simulink model "filtering"  (R2024a)
settings: Solver=FixedStepAuto  StartTime=0.0  StopTime=inf  FixedStep=1e-3  RelTol=1e-3
values from neighbouring files (symbols this model uses):
  net = trainNetwork(XTrain, YTrain, layers, options)    [lstm_ex.m]    (also in optimization.m; simpleCanvas.m)
undefined symbols (not defined in the file or in its folder): CR, LF
libraries: dspstat3 x5, instrumentseriallib x2, dspfdesign x1, deeplib x1
settings Model: Creator=samet  LastModifiedBy=samet
settings OptimizationCC: BlockReduction=off  DefaultParameterBehavior=Inlined  BufferReuse=off

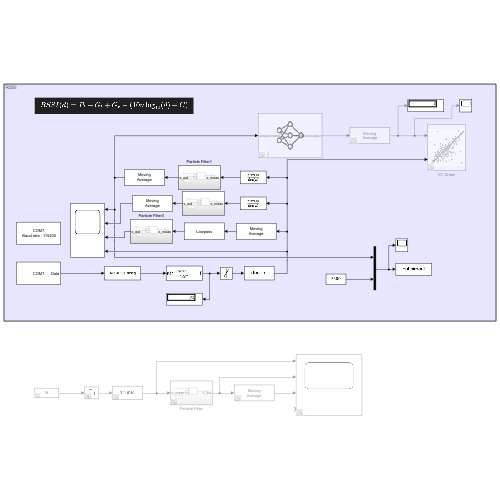
[thumbnail: Simulink's stored preview of the top-level diagram]
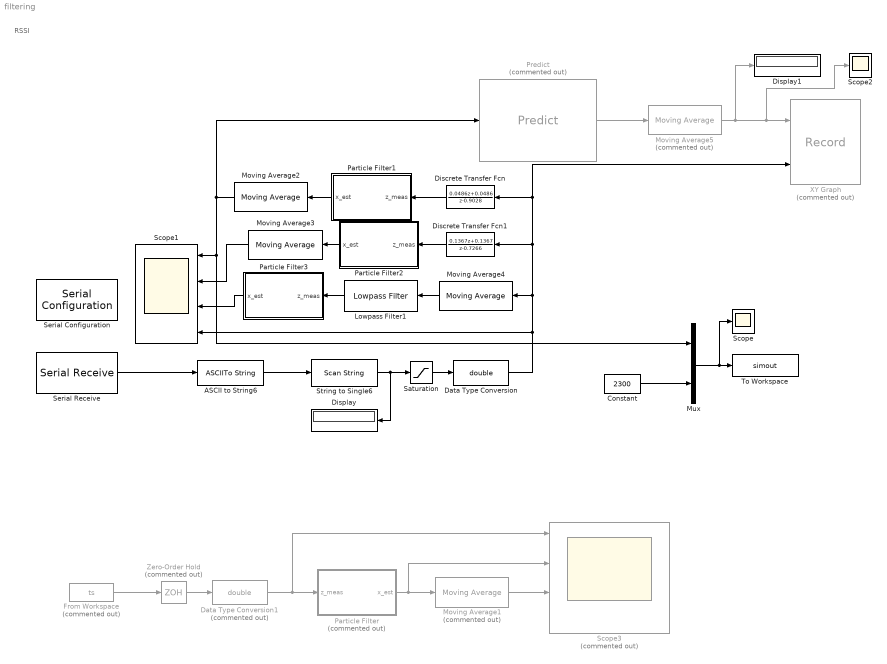
== system filtering ==
  note: RSSI
  ASCII to String6 : ASCIIToString
  Constant : Constant  Value=2300
  Data Type Conversion : DataTypeConversion  OutDataTypeStr=double  SaturateOnIntegerOverflow=off  RndMeth=Floor
  Data Type Conversion1 : DataTypeConversion  Commented=on  OutDataTypeStr=double  SaturateOnIntegerOverflow=off  RndMeth=Floor
  Discrete Transfer Fcn : DiscreteTransferFcn  Numerator=[0.0486 0.0486]  Denominator=[1 -0.9028]
  Discrete Transfer Fcn1 : DiscreteTransferFcn  Numerator=[0.1367 0.1367]  Denominator=[1 -0.7266]
  Display : Display
  Display1 : Display
  From Workspace : FromWorkspace  Commented=on  VariableName=ts
  Lowpass Filter1 : dspfdesign/Lowpass Filter  FilterType=FIR  DesignForMinimumOrder=on  FilterOrder=50  PassbandFrequency=8e3  StopbandFrequency=12e3  PassbandRipple=0.1  StopbandAttenuation=1  SampleRateMode=Specify on dialog  SampleRate=44100  SimulateUsing=Interpreted execution  roundingMode=Floor  coeffsDataTypeStr=fixdt(1,16)
  Moving Average1 : dspstat3/Moving Average  Commented=on  Method=Sliding window  ForgettingFactorPort=off  SpecifyWindowLength=on  WindowLength=4  OverlapLength=3  AllowArbitraryInputLength=off  ForgettingFactor=0.9  SimulateUsing=Interpreted execution
  Moving Average2 : dspstat3/Moving Average  Method=Sliding window  ForgettingFactorPort=off  SpecifyWindowLength=on  WindowLength=12  OverlapLength=11  AllowArbitraryInputLength=off  ForgettingFactor=0.9  SimulateUsing=Interpreted execution
  Moving Average3 : dspstat3/Moving Average  Method=Sliding window  ForgettingFactorPort=off  SpecifyWindowLength=on  WindowLength=12  OverlapLength=11  AllowArbitraryInputLength=off  ForgettingFactor=0.9  SimulateUsing=Interpreted execution
  Moving Average4 : dspstat3/Moving Average  Method=Sliding window  ForgettingFactorPort=off  SpecifyWindowLength=on  WindowLength=4  OverlapLength=3  AllowArbitraryInputLength=off  ForgettingFactor=0.9  SimulateUsing=Interpreted execution
  Moving Average5 : dspstat3/Moving Average  Commented=on  Method=Sliding window  ForgettingFactorPort=off  SpecifyWindowLength=on  WindowLength=12  OverlapLength=11  AllowArbitraryInputLength=off  ForgettingFactor=0.9  SimulateUsing=Interpreted execution
  Mux : Mux  Inputs=2
  Particle Filter : Subsystem  Commented=on
  Particle Filter1 : Subsystem
  Particle Filter2 : Subsystem
  Particle Filter3 : Subsystem
  Predict : deeplib/Predict  Commented=on  Network=Network from MAT-file  NetworkFunction=squeezenet  NetworkFilePath=C:\Users\samet\Desktop\net.mat  MiniBatchSize=128  InputDataFormats={'',''}  Predictions=on  Activations={}  ForceInterpretedSim=off  EnableDLNetwork=on  LastKnownNetworkFilePath=''  LastKnownNetworkTimeStamp=''
  Saturation : Saturate  UpperLimit=0  LowerLimit=-80
  Scope : Scope
  Scope1 : Scope  NumInputPorts=4
  Scope2 : Scope
  Scope3 : Scope  Commented=on  NumInputPorts=4
  Serial Configuration : instrumentseriallib/Serial Configuration  Priority=-200000  PortSel=COM7  Port=COM7  ComPort=COM7  BaudRate=115200  DataBits=8  Parity=none  StopBits=1  ByteOrder=little-endian  FlowControl=none  Timeout=10  SimulateUsing=Interpreted execution  BlockInModel=on  aMode=1
      settings: LibrarySourceBlock=embeddedtargetslib/Host Communication/Serial Configuration
  Serial Receive : instrumentseriallib/Serial Receive  Priority=1  PortSel=COM7  Port=COM7  ComPort=COM7  DataType=uint8  SaveDataType=uint8  ToggleHeader=off  Header=[]  ToggleDataSize=on  DataSize=[1 3]  ToggleTerminator=on  Terminator=CR/LF ('\r\n')  CustomTerminator='\n\r'  InputFormat=Row major  EnableBlockingMode=on  ActionDataUnavailable=Output last received value  ActionWhenDataUnavailable=Output last received value  CustomValue=0  SampleTime=0.01  SimulateUsing=Interpreted execution  BlockInModel=on  aMode=1
      settings: LibrarySourceBlock=embeddedtargetslib/Host Communication/Serial Receive
  String to Single6 : ScanString  Format="\"%f\""
  To Workspace : ToWorkspace  VariableName=simout  SampleTime=-1
      settings: Save2DSignal=2-D array (concatenate along first dimension)
  XY Graph : Record  Commented=on  FileSettingsInternal="{\"entries\":[{\"content\":{\"excelSettings\":{\"content\":{},\"type\":\"Streamout.ExcelSettings\"}},\"type\":\"Streamout.FileSettingStorage\",\"uuid\":\"\"}],\"packageUris\":[\"http:\\/\\/schema.mathworks.com\\/mf0\\/streamout_blocks\\/R2020a\"],\"version\":\"1.0\"}"  Layout=[1 1]  SignalsInternal="{\"entries\":[{\"content\":{\"signals\":[{\"content\":{\"blockPath\":[],\"dimensions\":[1,1],\"domain\":\"\",\"lineColor\":\"#22b573\",\"lineWidth\":2,\"port\":1,\"signalID\":1,\"signalName\":\"Moving\\nAverage5\"},\"type\":\"RecordBlkView.Signal\",\"uuid\":\"\"},{\"content\":{\"blockPath\":[],\"dimensions\":[1],\"domain\":\"\",\"lineColor\":\"#0072bd\",\"lineWidth\":2,\"port\":2,\"signalID\":2,\"signalName\":\"Data Type Conversion\"},\"type\":\"RecordBlkView.Signal\",\"uuid\":\"\"}]},\"type\":\"RecordBlkView.InputSignals\",\"uuid\":\"\"}],\"packageUris\":[\"http:\\/\\/schema.mathworks.com\\/mf0\\/streamout_blocks\\/R2020a\"],\"version\":\"1.0\"}"  VisualizationBindings="{\"xyplotplugin\":{\"info\":[{\"series\":[],\"subplotID\":1}]}}"  CompatibilityTag=XY
  Zero-Order Hold : ZeroOrderHold  Commented=on
  wires:
  ASCII to String6/1 -> String to Single6/1
  Serial Receive/1 -> ASCII to String6/1
  Mux/1 -> Scope/1, To Workspace/1
  String to Single6/1 -> Saturation/1, Display/1
  From Workspace/1 -> Zero-Order Hold/1
  Zero-Order Hold/1 -> Data Type Conversion1/1
  Data Type Conversion1/1 -> Scope3/1, Particle Filter/1(z_meas)
  Particle Filter/1(x_est) -> Scope3/2, Moving Average1/1
  Moving Average1/1 -> Scope3/3
  Constant/1 -> Mux/2
  Saturation/1 -> Data Type Conversion/1
  Predict/1 -> Moving Average5/1
  Data Type Conversion/1 -> Discrete Transfer Fcn/1, XY Graph/2, Discrete Transfer Fcn1/1, Moving Average4/1, Scope1/4
  Particle Filter2/1(x_est) -> Moving Average3/1
  Moving Average3/1 -> Scope1/2
  Moving Average4/1 -> Lowpass Filter1/1
  Lowpass Filter1/1 -> Particle Filter3/1(z_meas)
  Particle Filter3/1(x_est) -> Scope1/3
  Discrete Transfer Fcn/1 -> Particle Filter1/1(z_meas)
  Particle Filter1/1(x_est) -> Moving Average2/1
  Moving Average2/1 -> Predict/1, Mux/1, Scope1/1
  Discrete Transfer Fcn1/1 -> Particle Filter2/1(z_meas)
  Moving Average5/1 -> Scope2/1, XY Graph/1, Display1/1

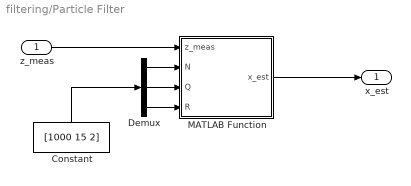
== system filtering/Particle Filter ==
  z_meas : Inport
  Constant : Constant  Value=[1000 15 2]
  Demux : Demux  Outputs=3
  MATLAB Function : MATLAB Function  TreatAsAtomicUnit=on
  x_est : Outport
  wires:
  Demux/2 -> MATLAB Function/3(Q)
  Demux/3 -> MATLAB Function/4(R)
  z_meas/1 -> MATLAB Function/1(z_meas)
  Demux/1 -> MATLAB Function/2(N)
  MATLAB Function/1(x_est) -> x_est/1
  Constant/1 -> Demux/1

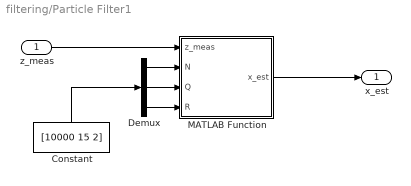
== system filtering/Particle Filter1 ==
  z_meas : Inport
  Constant : Constant  Value=[10000 15 2]
  Demux : Demux  Outputs=3
  MATLAB Function : MATLAB Function  TreatAsAtomicUnit=on
  x_est : Outport
  wires:
  Constant/1 -> Demux/1
  MATLAB Function/1(x_est) -> x_est/1
  Demux/1 -> MATLAB Function/2(N)
  z_meas/1 -> MATLAB Function/1(z_meas)
  Demux/3 -> MATLAB Function/4(R)
  Demux/2 -> MATLAB Function/3(Q)

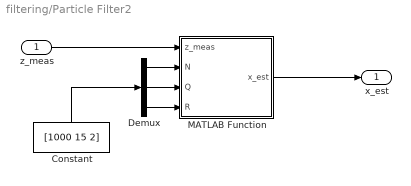
== system filtering/Particle Filter2 ==
  z_meas : Inport
  Constant : Constant  Value=[1000 15 2]
  Demux : Demux  Outputs=3
  MATLAB Function : MATLAB Function  TreatAsAtomicUnit=on
  x_est : Outport
  wires:
  Demux/2 -> MATLAB Function/3(Q)
  Demux/3 -> MATLAB Function/4(R)
  z_meas/1 -> MATLAB Function/1(z_meas)
  Demux/1 -> MATLAB Function/2(N)
  MATLAB Function/1(x_est) -> x_est/1
  Constant/1 -> Demux/1

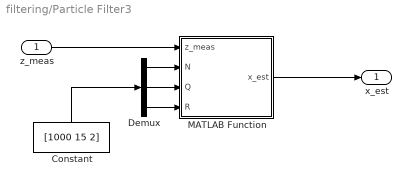
== system filtering/Particle Filter3 ==
  z_meas : Inport
  Constant : Constant  Value=[1000 15 2]
  Demux : Demux  Outputs=3
  MATLAB Function : MATLAB Function  TreatAsAtomicUnit=on
  x_est : Outport
  wires:
  Demux/2 -> MATLAB Function/3(Q)
  Demux/3 -> MATLAB Function/4(R)
  z_meas/1 -> MATLAB Function/1(z_meas)
  Demux/1 -> MATLAB Function/2(N)
  MATLAB Function/1(x_est) -> x_est/1
  Constant/1 -> Demux/1

== matlab function filtering/Particle Filter/MATLAB Function ==
  data: z_meas input; x_est output; N input; Q input; R input
function x_est = particle_filter(z_meas, N, Q, R)
    persistent particles weights init;
    if isempty(init)
        particles = randn(N, 1) * 5;  
        weights = ones(N, 1) / N;
        init = true;
    end

    % 1. Parçacıkları Güncelle (Durum Geçişi)
    particles = particles + sqrt(Q) * randn(N, 1);

    % 2. Ölçüm Güncellemesi
    weights = exp(-0.5 * ((z_meas - particles).^2) / R);
    weights = weights / sum(weights);

    % 3. Tahmini Hesapla
    x_est = sum(weights .* particles);

    % 4. Resampling (Yeniden Örnekleme)
    Neff = 1 / sum(weights.^2);
    if Neff < N / 2
        indices = randsample(N, N, true, weights);
        particles = particles(indices);
        weights = ones(N, 1) / N;
    end
end

== matlab function filtering/Particle Filter1/MATLAB Function ==
  data: z_meas input; x_est output; N input; Q input; R input
function x_est = particle_filter(z_meas, N, Q, R)
    persistent particles weights init;
    if isempty(init)
        particles = randn(N, 1) * 5;  
        weights = ones(N, 1) / N;
        init = true;
    end

    % 1. Parçacıkları Güncelle (Durum Geçişi)
    particles = particles + sqrt(Q) * randn(N, 1);

    % 2. Ölçüm Güncellemesi
    weights = exp(-0.5 * ((z_meas - particles).^2) / R);
    weights = weights / sum(weights);

    % 3. Tahmini Hesapla
    x_est = sum(weights .* particles);

    % 4. Resampling (Yeniden Örnekleme)
    Neff = 1 / sum(weights.^2);
    if Neff < N / 2
        indices = randsample(N, N, true, weights);
        particles = particles(indices);
        weights = ones(N, 1) / N;
    end
end

== matlab function filtering/Particle Filter2/MATLAB Function ==
  data: z_meas input; x_est output; N input; Q input; R input
function x_est = particle_filter(z_meas, N, Q, R)
    persistent particles weights init;
    if isempty(init)
        particles = randn(N, 1) * 5;  
        weights = ones(N, 1) / N;
        init = true;
    end

    % 1. Parçacıkları Güncelle (Durum Geçişi)
    particles = particles + sqrt(Q) * randn(N, 1);

    % 2. Ölçüm Güncellemesi
    weights = exp(-0.5 * ((z_meas - particles).^2) / R);
    weights = weights / sum(weights);

    % 3. Tahmini Hesapla
    x_est = sum(weights .* particles);

    % 4. Resampling (Yeniden Örnekleme)
    Neff = 1 / sum(weights.^2);
    if Neff < N / 2
        indices = randsample(N, N, true, weights);
        particles = particles(indices);
        weights = ones(N, 1) / N;
    end
end

== matlab function filtering/Particle Filter3/MATLAB Function ==
  data: z_meas input; x_est output; N input; Q input; R input
function x_est = particle_filter(z_meas, N, Q, R)
    persistent particles weights init;
    if isempty(init)
        particles = randn(N, 1) * 5;  
        weights = ones(N, 1) / N;
        init = true;
    end

    % 1. Parçacıkları Güncelle (Durum Geçişi)
    particles = particles + sqrt(Q) * randn(N, 1);

    % 2. Ölçüm Güncellemesi
    weights = exp(-0.5 * ((z_meas - particles).^2) / R);
    weights = weights / sum(weights);

    % 3. Tahmini Hesapla
    x_est = sum(weights .* particles);

    % 4. Resampling (Yeniden Örnekleme)
    Neff = 1 / sum(weights.^2);
    if Neff < N / 2
        indices = randsample(N, N, true, weights);
        particles = particles(indices);
        weights = ones(N, 1) / N;
    end
end
